simulink model "NonlinearPassiveObserver"  (R2023a)
settings: Solver=VariableStepAuto  StartTime=0.0  StopTime=10.0  RelTol=1e-3
values from neighbouring files (symbols this model uses):
  C_w = [zeros(3,3) eye(3)]    [CPM.m]    (also in control_plant_model.m; init.m)
  D = [-Xu 0 0 ... (first row only)    [CPM.m]    (also in control_plant_model.m; init.m = [2.6486e5 0 0)
  K1 = [diag([k1, k2, k3]) ... (first row only)    [init.m]
  K2 = diag([k7, k8, k9])    [init.m]
  K3 = 0.08 * K4    [init.m]
  K4 = 2.5e-1*diag([k13, k14, k15])    [init.m]
  M_inv = inv(M)    [CPM.m]    (also in ekf_script.m = model.M_inv; init.m)
  T_b = diag([1 1 1])    [CPM.m]    (also in control_plant_model.m; init.m = 60*diag([1 1 1]))
libraries: marine_gnc x3
settings Model: Creator=33769  LastModifiedBy=33769

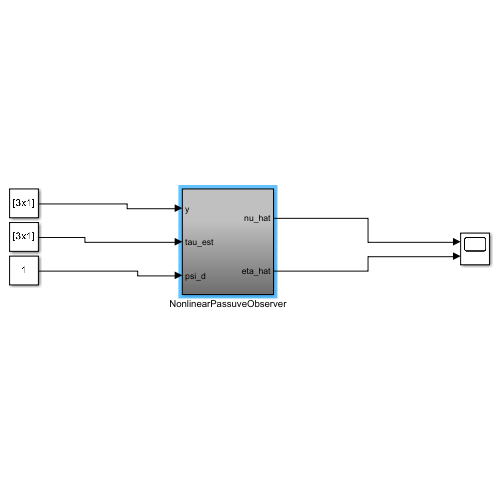
[thumbnail: Simulink's stored preview of the top-level diagram]
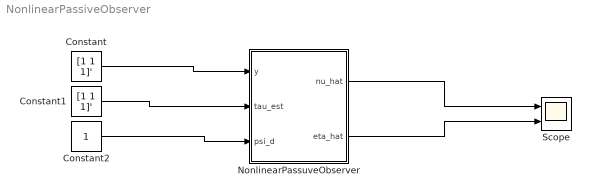
== system NonlinearPassiveObserver ==
  Constant : Constant  Value=[1 1 1]'
  Constant1 : Constant  Value=[1 1 1]'
  Constant2 : Constant
  NonlinearPassuveObserver : Subsystem
  Scope : Scope  NumInputPorts=2
  wires:
  Constant1/1 -> NonlinearPassuveObserver/2(tau_est)
  Constant/1 -> NonlinearPassuveObserver/1(y)
  Constant2/1 -> NonlinearPassuveObserver/3(psi_d)
  NonlinearPassuveObserver/1(nu_hat) -> Scope/1
  NonlinearPassuveObserver/2(eta_hat) -> Scope/2

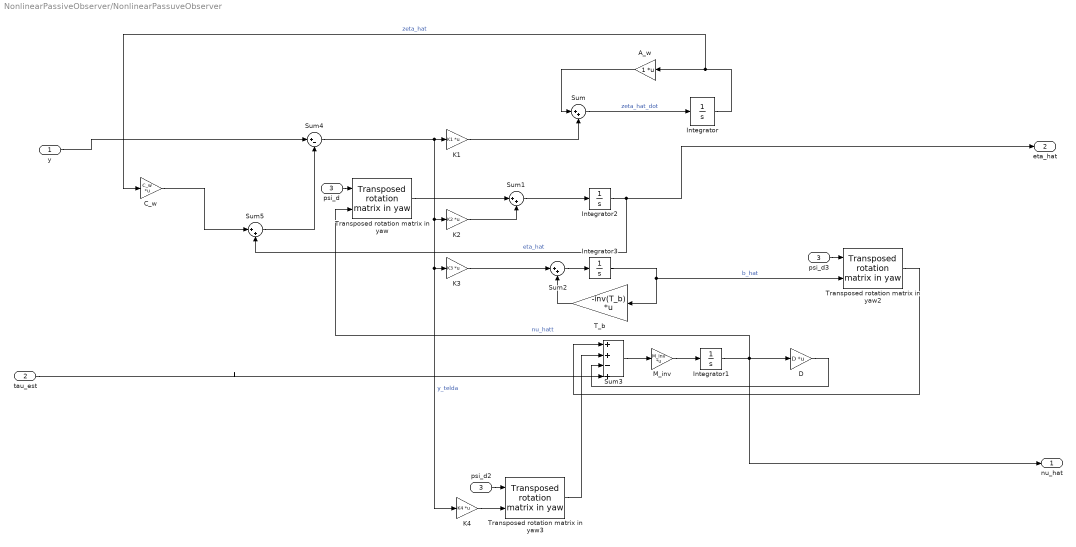
== system NonlinearPassiveObserver/NonlinearPassuveObserver ==
  y : Inport
  tau_est : Inport  Port=2
  psi_d : Inport  Port=3
  A_w : Gain  Multiplication=Matrix(K*u)
  C_w : Gain  Gain=C_w  Multiplication=Matrix(K*u)
  D : Gain  Gain=D  Multiplication=Matrix(K*u)
  Integrator{,1..3} (4 alike) : Integrator
  K1 : Gain  Gain=K1  Multiplication=Matrix(K*u)
  K2 : Gain  Gain=K2  Multiplication=Matrix(K*u)
  K3 : Gain  Gain=K3  Multiplication=Matrix(K*u)
  K4 : Gain  Gain=K4  Multiplication=Matrix(K*u)
  M_inv : Gain  Gain=M_inv  Multiplication=Matrix(K*u)
  Sum{,1..2,5} (4 alike) : Sum  Inputs=|++
  Sum3 : Sum  Inputs=|++-+
  Sum4 : Sum  Inputs=|+-
  T_b : Gain  Gain=-inv(T_b)  Multiplication=Matrix(K*u)
  Transposed rotation matrix in yaw : marine_gnc/Models/ Kinematics/Transposed rotation  matrix in yaw
  Transposed rotation matrix in yaw2 : marine_gnc/Models/ Kinematics/Transposed rotation  matrix in yaw
  Transposed rotation matrix in yaw3 : marine_gnc/Models/ Kinematics/Transposed rotation  matrix in yaw
  psi_d2 : InportShadow  Port=3
  psi_d3 : InportShadow  Port=3
  nu_hat : Outport  VectorParamsAs1DForOutWhenUnconnected=off
  eta_hat : Outport  Port=2  VectorParamsAs1DForOutWhenUnconnected=off
  wires:
  Sum4/1 -> K1/1, K2/1, K3/1, K4/1  "y_telda"
  Sum/1 -> Integrator/1  "zeta_hat_dot"
  Integrator1/1 -> D/1, nu_hat/1, Transposed rotation matrix in yaw/2  "nu_hatt"
  Integrator3/1 -> T_b/1, Transposed rotation matrix in yaw2/2  "b_hat"
  Transposed rotation matrix in yaw/1 -> Sum1/1
  K2/1 -> Sum1/2
  Sum1/1 -> Integrator2/1
  Sum2/1 -> Integrator3/1
  T_b/1 -> Sum2/2
  K3/1 -> Sum2/1
  Transposed rotation matrix in yaw2/1 -> Sum3/1
  K4/1 -> Transposed rotation matrix in yaw3/2
  M_inv/1 -> Integrator1/1
  Sum3/1 -> M_inv/1
  Integrator2/1 -> eta_hat/1, Sum5/2  "eta_hat"
  y/1 -> Sum4/1
  C_w/1 -> Sum5/1
  Sum5/1 -> Sum4/2
  K1/1 -> Sum/2
  psi_d/1 -> Transposed rotation matrix in yaw/1
  psi_d2/1 -> Transposed rotation matrix in yaw3/1
  psi_d3/1 -> Transposed rotation matrix in yaw2/1
  Transposed rotation matrix in yaw3/1 -> Sum3/2
  tau_est/1 -> Sum3/4
  D/1 -> Sum3/3
  Integrator/1 -> C_w/1, A_w/1  "zeta_hat"
  A_w/1 -> Sum/1
